simulink model "Test_Maps"  (R2018b)
settings: Solver=VariableStepAuto  StartTime=0.0  StopTime=time_dist(end)  RelTol=1e-3
undefined symbols (not defined in the file or in its folder): BC_dist, CS_dist, time_dist
libraries: platooning_custom_blocks x1
settings Model: Creator=Aman-Home  LastModifiedBy=Aman-Home

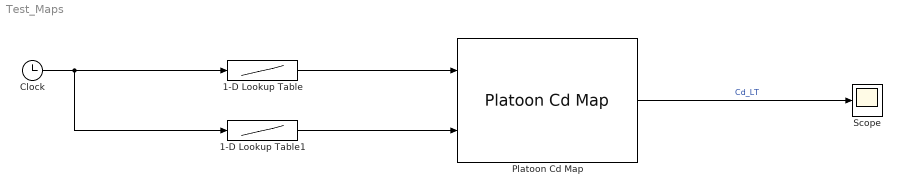
== system Test_Maps ==
  1-D Lookup Table : Lookup_n-D  NumberOfTableDimensions=1  BreakpointsForDimension1=time_dist  Table=BC_dist  InternalRulePriority=Speed  RndMeth=Simplest  InputSameDT=on
  1-D Lookup Table1 : Lookup_n-D  NumberOfTableDimensions=1  BreakpointsForDimension1=time_dist  Table=CS_dist  InternalRulePriority=Speed  RndMeth=Simplest  InputSameDT=on
  Clock : Clock
      settings: Decimation=100
  Platoon Cd Map : platooning_custom_blocks/Platoon Cd Map  msk_platoon_type=Three Truck  pos=Lead  msk_platoon_cd_map=Cd_Map  msk_platoon_cd_map_t2=Cd_Map_T2  msk_d1_bpt=d_11  msk_d2_bpt=d_22  msk_cd_avg=0.52
  Scope : Scope
  wires:
  1-D Lookup Table/1 -> Platoon Cd Map/1
  1-D Lookup Table1/1 -> Platoon Cd Map/2
  Platoon Cd Map/1 -> Scope/1  "Cd_LT"
  Clock/1 -> 1-D Lookup Table1/1, 1-D Lookup Table/1
